simulink model "minimal"  (R2015a)
settings: Solver=ode45  StartTime=0.0  StopTime=10.0  RelTol=1e-3
values from neighbouring files (symbols this model uses):
  K = dlqr(alpha*Phi_aug, alpha*Gamma_aug, Q, R)    [double_lqg.m]    (also in load_control.m; load_single_lqg.m = place(params.Phi, params.Gamma, c_z_poles); main.m = dlqr(Phi, Gamma, Q, R); run_design.m = dlqr(Phi, Gamma, Q, R))
  params = catstruct(params, sys.params_str)    [double_lqg.m]    (also in load_mechanism_params.m = params(1:13); load_params.m = [g, m0, b0,                m1, I1, b1, L1, L1_cg,           ; load_single_mechanism_params.m = params(1:8); load_single_params.m = [g, m0, b0,                m1, I1, b1, L1, L1_cg,           )
settings Model: Creator=BPeixoto  LastModifiedBy=BPeixoto

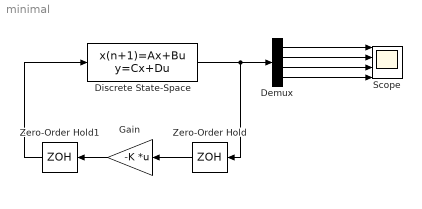
== system minimal ==
  Demux : Demux
  Discrete State-Space : DiscreteStateSpace  A=params.Phi  B=params.Gamma  C=params.C  D=params.D_  X0=[params.q0, params.qp0].'  SampleTime=params.ts
  Gain : Gain  Gain=-K  Multiplication=Matrix(K*u) (u vector)
  Scope : Scope  NumInputPorts=4
      settings: YMin=-5~-5~-5~-5  YMax=5~5~5~5
  Zero-Order Hold : ZeroOrderHold  SampleTime=params.ts
  Zero-Order Hold1 : ZeroOrderHold  SampleTime=params.ts
  wires:
  Discrete State-Space/1 -> Zero-Order Hold/1, Demux/1
  Demux/3 -> Scope/3
  Demux/4 -> Scope/4
  Demux/1 -> Scope/1
  Demux/2 -> Scope/2
  Gain/1 -> Zero-Order Hold1/1
  Zero-Order Hold1/1 -> Discrete State-Space/1
  Zero-Order Hold/1 -> Gain/1
